simulink model "px4demo_serial"  (R2019b)
settings: Solver=FixedStepAuto  StartTime=0.0  StopTime=inf  RelTol=1e-3  EnableMultiTasking=on
libraries: px4lib x3, simulink x1, px4Sensorslib x1
settings Model: ExtModeTrigDuration=10  Creator=The MathWorks, Inc.  LastModifiedBy=The MathWorks, Inc.
settings SolverCC: PositivePriorityOrder=on
settings OptimizationCC: EnhancedBackFolding=on  PassReuseOutputArgsAs=Individual arguments  ZeroExternalMemoryAtStartup=off  ZeroInternalMemoryAtStartup=off  MaxStackSize=64  OptimizeBlockOrder=speed  DifferentSizesBufferReuse=on  OptimizationCustomize=off  EfficientTunableParamExpr=on
settings DebuggingCC: InheritedTsInSrcMsg=none  ParameterTunabilityLossMsg=error
settings HardwareCC: ProdBitPerPointer=32  ProdBitPerSizeT=32  ProdBitPerPtrDiffT=32  ProdLargestAtomicInteger=Long  ProdLargestAtomicFloat=Double  ProdWordSize=32  ProdLongLongMode=on  ProdHWDeviceType=ARM Compatible->ARM Cortex
settings SFSimCC: MATLABDynamicMemAlloc=off
settings RTWCC: SystemTargetFile=ert.tlc  HardwareBoard=PX4 Pixhawk Series  TLCOptions="-aInlineSetEventsForThisBaseRateFcn=TLC_FALSE -aSuppressMultiTaskScheduler=TLC_FALSE  -aRateBasedStepFcn=0"  TemplateMakefile=ert_default_tmf  Toolchain=GNU Tools for PX4 Autopilots  IncludeHyperlinkInReport=on  TargetLang=C++
settings CodeAppCC: ForceParamTrailComments=on  IgnoreCustomStorageClasses=off  OperatorAnnotations=on  SimulinkDataObjDesc=on  SFDataObjDesc=on  InsertBlockDesc=on
settings ERTTargetCC: SupportVariableSizeSignals=on

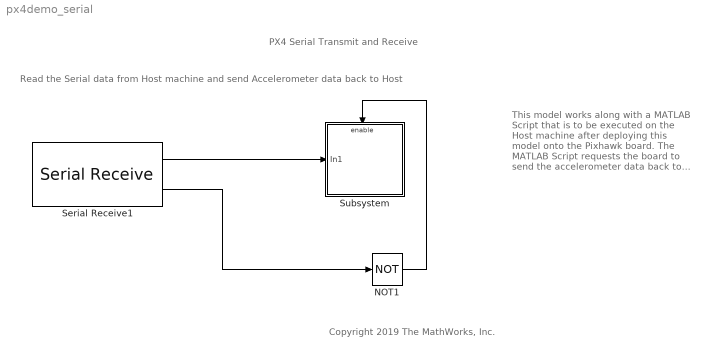
== system px4demo_serial ==
  note: Read the Serial data from Host machine and send Accelerometer data back to
      | Host
  note: PX4 Serial Transmit and Receive
  note: Copyright 2019 The MathWorks, Inc.
  note: This model works along with a MATLAB Script that is to be executed on the Host machine after deploying this model onto the Pixhawk board.
      |
      | The MATLAB Script requests the board to send the accelerometer data back to the host.
  NOT1 : Logic  Operator=NOT  IconShape=distinctive  AllPortsSameDT=off  OutDataTypeStr=boolean
  Serial Receive1 : px4lib/Serial Receive  SCIModule=/dev/ttyACM0  DataType=uint8  DataLength=10  OutputStatus=on  SampleTime=0.1  BlockingMode=off  PartialData=off  Timeout=5
      settings: SourceProductName=Embedded Coder Support Package for PX4 Autopilots  SourceProductBaseCode=PX4AUTOPILOTS
  Subsystem : Subsystem
  wires:
  Serial Receive1/2 -> NOT1/1
  Serial Receive1/1 -> Subsystem/1(In1)
  NOT1/1 -> Subsystem/Enable

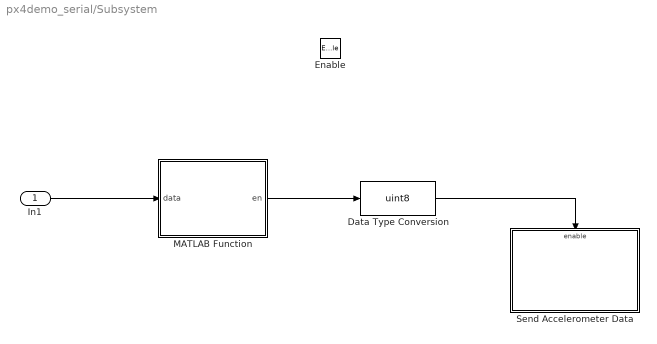
== system px4demo_serial/Subsystem ==
  In1 : Inport
  Enable : EnablePort
  Data Type Conversion : DataTypeConversion  OutDataTypeStr=uint8
  MATLAB Function : MATLAB Function  TreatAsAtomicUnit=on
  Send Accelerometer Data : Subsystem
  wires:
  In1/1 -> MATLAB Function/1(data)
  MATLAB Function/1(en) -> Data Type Conversion/1
  Data Type Conversion/1 -> Send Accelerometer Data/Enable

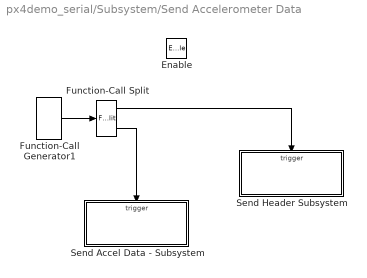
== system px4demo_serial/Subsystem/Send Accelerometer Data ==
  Enable : EnablePort
  Function-Call Generator1 : simulink/Ports & Subsystems/Function-Call Generator  sample_time=-1  numberOfIterations=1
  Function-Call Split : FunctionCallSplit  IconShape=distinctive  NumOutputPorts=2  OutputPortLayout=default
  Send Accel Data - Subsystem : Subsystem  TreatAsAtomicUnit=on
  Send Header Subsystem : Subsystem  TreatAsAtomicUnit=on
  wires:
  Function-Call Generator1/1 -> Function-Call Split/1
  Function-Call Split/1 -> Send Header Subsystem/Trigger
  Function-Call Split/2 -> Send Accel Data - Subsystem/Trigger

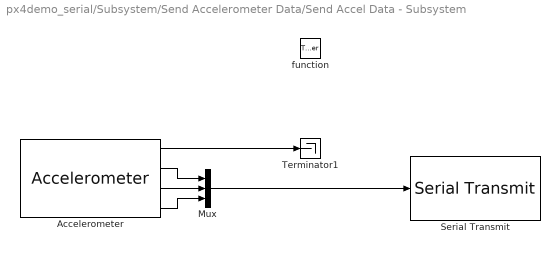
== system px4demo_serial/Subsystem/Send Accelerometer Data/Send Accel Data - Subsystem ==
  function : TriggerPort  TriggerType=function-call  VariantControl=Variant
  Accelerometer : px4Sensorslib/Accelerometer  uorbTimeStamp=off  BlockingMode=off  BlockTimeout=1e-3  sampleTime=-1
      settings: SourceProductName=Embedded Coder Support Package for PX4 Autopilots  SourceProductBaseCode=PX4AUTOPILOTS
  Mux : Mux  Inputs=3
  Serial Transmit : px4lib/Serial Transmit  SCIModule=/dev/ttyACM0
      settings: SourceProductName=Embedded Coder Support Package for PX4 Autopilots  SourceProductBaseCode=PX4AUTOPILOTS
  Terminator1 : Terminator
  wires:
  Mux/1 -> Serial Transmit/1
  Accelerometer/1 -> Terminator1/1
  Accelerometer/2 -> Mux/1
  Accelerometer/3 -> Mux/2
  Accelerometer/4 -> Mux/3

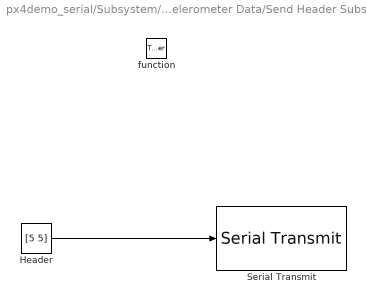
== system px4demo_serial/Subsystem/Send Accelerometer Data/Send Header Subsystem ==
  function : TriggerPort  TriggerType=function-call  VariantControl=Variant
  Header : Constant  Value=[5 5]  OutDataTypeStr=uint8  SampleTime=-1
  Serial Transmit : px4lib/Serial Transmit  SCIModule=/dev/ttyACM0
      settings: SourceProductName=Embedded Coder Support Package for PX4 Autopilots  SourceProductBaseCode=PX4AUTOPILOTS
  wires:
  Header/1 -> Serial Transmit/1

== matlab function px4demo_serial/Subsystem/MATLAB Function ==
  data: data input; en output
% PARSERECEIVEDDATA

%This function is executed only when valid serial data of 10 * 1 uint8
%data is received. This parses the data and if it is valid, sets a flag
%which is used by the downstream Enabled subsystem block to send
%accelerometer data back to the host requesting it.

% Copyright 2019 The MathWorks, Inc.
function en  = parseReceivedData(data)

%Initialize the variables
data = data';
packet = uint8(zeros(1,3));
packetfound = false;

%signaturePacket denotes the expected packet. If the data received matches
%this, it is considered as a valid request for the Pixhawk board to send
%Accelerometer data
signaturePacket = uint8([9 9 9]);
header = [7 7];

len = length(header);

% First, find possible header start locations; i.e., match the first element in the
% header.
start = find(data==header(1));

% Next remove start values that are too close to the end to possibly match
% the header.
endVals = start+len-1;
start(endVals>length(data)) = [];

% Next, loop over elements of header, usually much shorter than length of
% array, to check which possible header start locations are valid still.
for pattval = 2:len
    % check viable locations in array
    locs = header(pattval) == data(start+pattval-1);
    % delete false ones from indices
    start(~locs) = [];
end

%Packet = Data - Header
expectedPacketSize = len + length(signaturePacket);

if ~isempty(start)
    for i = 1:length(start)
        %Verify if the size of data between 2 consecutive header start
        %indices is equal to the expectedPacketSize
        if isequal(start(i+1)-start(i),expectedPacketSize)
            
            %Extract the packet by stripping the header from the data
            packet = data(start(i)+len:start(i+1)-1);
            if ~isequal(length(packet),(expectedPacketSize-len))
                error('ERROR:Wrong packet size');
            end
            
            %Once a valid packet is found, exit the for loop
            packetfound = true;
            break;
        else
            continue
        end
    end
else
    packetfound = false;
end

%The downstream enabled subsystem uses this en flag
if packetfound && isequal(packet,signaturePacket)
    %Set the flag only if the received packet matches the expected
    %signature packet
    en = 1;
else
    en = 0;
end

end
